simulink model "MIL4L3_SW6_V1_20220211"  (R2018b)
settings: Solver=FixedStepAuto  StartTime=0.0  StopTime=inf  FixedStep=0.001  RelTol=1e-3
PreLoadFcn:
  | A0_MILtest;
undefined symbols (not defined in the file or in its folder): Clb_ICADirect_LaneDisp_StateFive, Clb_ICADirect_LaneDisp_StateFour, Clb_ICADirect_LaneDisp_StateOne, Clb_ICADirect_LaneDisp_StateThree, Clb_ICADirect_LaneDisp_StateTwo, Clb_ICADirect_LaneDisp_StateZero, Clb_ICADirect_LaneDispSW, Clb_ICADirect_TrnLghtsCom_Switch, Clb_ICADirect_TrnLghtsCom_Value, Clb_ICADirect_TrnLghtsCrtl_Inhb, IMAP_Clb_ACU_Driver_Belt, IMAP_Clb_ACU_Driver_Belt_Over, IMAP_Clb_ACU_Passenger_Belt, IMAP_Clb_ACU_Passenger_Belt_Over, IMAP_Clb_ACU_RearLeft_Belt, IMAP_Clb_ACU_RearLeft_Belt_Over, IMAP_Clb_ACU_RearMiddle_Belt, IMAP_Clb_ACU_RearMiddle_Belt_Over, IMAP_Clb_ACU_RearRight_Belt, IMAP_Clb_ACU_RearRight_Belt_Over, IMAP_Clb_AEB_Switch, IMAP_Clb_AEB_Switch_Over, IMAP_Clb_ALC_TLC_Mode, IMAP_Clb_ALC_TLC_Mode_Over, IMAP_Clb_BCM_Battery_Voltage, IMAP_Clb_BCM_Battery_Voltage_Over, IMAP_Clb_BCM_BrakeLamp_State, IMAP_Clb_BCM_BrakeLamp_State_Over, IMAP_Clb_BCM_CHMSL_Status, IMAP_Clb_BCM_CHMSL_Status_Over, IMAP_Clb_BCM_Door_Lock_State, IMAP_Clb_BCM_Door_Lock_State_Over, IMAP_Clb_BCM_FrontWiper_State, IMAP_Clb_BCM_FrontWiper_State_Over, IMAP_Clb_BCM_FrontWiper_Switch, IMAP_Clb_BCM_FrontWiper_Switch_Over, IMAP_Clb_BCM_HazardLamp, IMAP_Clb_BCM_HazardLamp_Over, IMAP_Clb_BCM_HazardLamp_Switch, IMAP_Clb_BCM_HazardLamp_Switch_Over, IMAP_Clb_BCM_HighBeam_State, IMAP_Clb_BCM_HighBeam_State_Over, IMAP_Clb_BCM_Ignition_State, IMAP_Clb_BCM_Ignition_State_Over, IMAP_Clb_BCM_IHBC_Enabled, IMAP_Clb_BCM_IHBC_Enabled_Over, IMAP_Clb_BCM_Left_Light, IMAP_Clb_BCM_Left_Light_Over, IMAP_Clb_BCM_LeftTurn_Switch, IMAP_Clb_BCM_LeftTurn_Switch_Over, IMAP_Clb_BCM_LF_Door_State, IMAP_Clb_BCM_LF_Door_State_Over, IMAP_Clb_BCM_LowBeam_State, IMAP_Clb_BCM_LowBeam_State_Over, IMAP_Clb_BCM_LR_Door_State, IMAP_Clb_BCM_LR_Door_State_Over, IMAP_Clb_BCM_RF_Door_State, IMAP_Clb_BCM_RF_Door_State_Over, IMAP_Clb_BCM_Right_Light, IMAP_Clb_BCM_Right_Light_Over ... (+547)
libraries: CarMaker4SL x2153, simulink x292, dspstat3 x3, canmsglib x2, simulink_extras x1
(part 24 of 52)

== system MIL4L3_SW6_V1_20220211/CarMaker/VehicleControl/Data Inport/SDFA-L3/Subsystem215 ==
  BusCreator : BusCreator  Inputs=24
  Ground{,1..19} (20 alike) : Ground
  Read CM Dict : CarMaker4SL/Read CM Dict  xname=User.IO.Out.ObjectID_00  xsync=off
  Read CM Dict1 : CarMaker4SL/Read CM Dict  xname=User.IO.Out.ObjectID_01  xsync=off
  Read CM Dict2 : CarMaker4SL/Read CM Dict  xname=User.IO.Out.ObjectID_02  xsync=off
  Read CM Dict3 : CarMaker4SL/Read CM Dict  xname=User.IO.Out.ObjectID_03  xsync=off
  ObjectID : Outport
  wires:
  Ground12/1 -> BusCreator/21
  Ground16/1 -> BusCreator/19
  Ground14/1 -> BusCreator/17
  Ground2/1 -> BusCreator/7
  Read CM Dict1/1 -> BusCreator/2
  Ground6/1 -> BusCreator/11
  Read CM Dict2/1 -> BusCreator/3
  Ground10/1 -> BusCreator/15
  Read CM Dict/1 -> BusCreator/1
  Ground17/1 -> BusCreator/20
  Ground4/1 -> BusCreator/9
  Ground13/1 -> BusCreator/22
  Ground/1 -> BusCreator/5
  Ground1/1 -> BusCreator/6
  Ground15/1 -> BusCreator/18
  Ground7/1 -> BusCreator/12
  Ground8/1 -> BusCreator/13
  Ground11/1 -> BusCreator/16
  BusCreator/1 -> ObjectID/1
  Ground9/1 -> BusCreator/14
  Ground3/1 -> BusCreator/8
  Ground5/1 -> BusCreator/10
  Ground18/1 -> BusCreator/23
  Ground19/1 -> BusCreator/24
  Read CM Dict3/1 -> BusCreator/4

== system MIL4L3_SW6_V1_20220211/CarMaker/VehicleControl/Data Inport/SDFA-L3/Subsystem216 ==
  Bus Creator : BusCreator  Inputs=20
  Ground{,1..15} (16 alike) : Ground
  Read CM Dict : CarMaker4SL/Read CM Dict  xname=User.IO.Out.IFC_obj01_Width  xsync=off
  Read CM Dict1 : CarMaker4SL/Read CM Dict  xname=User.IO.Out.IFC_obj02_Width  xsync=off
  Read CM Dict2 : CarMaker4SL/Read CM Dict  xname=User.IO.Out.IFC_obj03_Width  xsync=off
  Read CM Dict3 : CarMaker4SL/Read CM Dict  xname=User.IO.Out.IFC_obj04_Width  xsync=off
  obj_Width : Outport
  wires:
  Bus Creator/1 -> obj_Width/1
  Ground15/1 -> Bus Creator/20
  Ground11/1 -> Bus Creator/16
  Ground14/1 -> Bus Creator/19
  Ground12/1 -> Bus Creator/17
  Ground3/1 -> Bus Creator/8
  Ground1/1 -> Bus Creator/6
  Read CM Dict1/1 -> Bus Creator/2
  Read CM Dict/1 -> Bus Creator/1
  Ground6/1 -> Bus Creator/11
  Ground10/1 -> Bus Creator/15
  Ground13/1 -> Bus Creator/18
  Ground2/1 -> Bus Creator/7
  Ground/1 -> Bus Creator/5
  Ground7/1 -> Bus Creator/12
  Read CM Dict3/1 -> Bus Creator/4
  Ground4/1 -> Bus Creator/9
  Ground9/1 -> Bus Creator/14
  Ground5/1 -> Bus Creator/10
  Ground8/1 -> Bus Creator/13
  Read CM Dict2/1 -> Bus Creator/3

== system MIL4L3_SW6_V1_20220211/CarMaker/VehicleControl/Data Inport/SDFA-L3/Subsystem217 ==
  Bus Creator : BusCreator  Inputs=20
  Ground{,1..15} (16 alike) : Ground
  Read CM Dict : CarMaker4SL/Read CM Dict  xname=User.IO.Out.IFC_obj01_TypeProb  xsync=off
  Read CM Dict1 : CarMaker4SL/Read CM Dict  xname=User.IO.Out.IFC_obj02_TypeProb  xsync=off
  Read CM Dict2 : CarMaker4SL/Read CM Dict  xname=User.IO.Out.IFC_obj03_TypeProb  xsync=off
  Read CM Dict3 : CarMaker4SL/Read CM Dict  xname=User.IO.Out.IFC_obj04_TypeProb  xsync=off
  obj_TypeProb : Outport
  wires:
  Bus Creator/1 -> obj_TypeProb/1
  Ground15/1 -> Bus Creator/20
  Ground11/1 -> Bus Creator/16
  Ground14/1 -> Bus Creator/19
  Ground12/1 -> Bus Creator/17
  Ground3/1 -> Bus Creator/8
  Ground1/1 -> Bus Creator/6
  Read CM Dict1/1 -> Bus Creator/2
  Read CM Dict/1 -> Bus Creator/1
  Ground6/1 -> Bus Creator/11
  Ground10/1 -> Bus Creator/15
  Ground13/1 -> Bus Creator/18
  Ground2/1 -> Bus Creator/7
  Ground/1 -> Bus Creator/5
  Ground7/1 -> Bus Creator/12
  Read CM Dict3/1 -> Bus Creator/4
  Ground4/1 -> Bus Creator/9
  Ground9/1 -> Bus Creator/14
  Ground5/1 -> Bus Creator/10
  Ground8/1 -> Bus Creator/13
  Read CM Dict2/1 -> Bus Creator/3

== system MIL4L3_SW6_V1_20220211/CarMaker/VehicleControl/Data Inport/SDFA-L3/Subsystem218 ==
  Bus Creator : BusCreator  Inputs=20
  Ground{,1..15} (16 alike) : Ground
  Read CM Dict : CarMaker4SL/Read CM Dict  xname=User.IO.Out.IFC_obj01_Height  xsync=off
  Read CM Dict1 : CarMaker4SL/Read CM Dict  xname=User.IO.Out.IFC_obj02_Height  xsync=off
  Read CM Dict2 : CarMaker4SL/Read CM Dict  xname=User.IO.Out.IFC_obj03_Height  xsync=off
  Read CM Dict3 : CarMaker4SL/Read CM Dict  xname=User.IO.Out.IFC_obj04_Height  xsync=off
  obj_Height : Outport
  wires:
  Bus Creator/1 -> obj_Height/1
  Ground15/1 -> Bus Creator/20
  Ground11/1 -> Bus Creator/16
  Ground14/1 -> Bus Creator/19
  Ground12/1 -> Bus Creator/17
  Ground3/1 -> Bus Creator/8
  Ground1/1 -> Bus Creator/6
  Read CM Dict1/1 -> Bus Creator/2
  Read CM Dict/1 -> Bus Creator/1
  Ground6/1 -> Bus Creator/11
  Ground10/1 -> Bus Creator/15
  Ground13/1 -> Bus Creator/18
  Ground2/1 -> Bus Creator/7
  Ground/1 -> Bus Creator/5
  Ground7/1 -> Bus Creator/12
  Read CM Dict3/1 -> Bus Creator/4
  Ground4/1 -> Bus Creator/9
  Ground9/1 -> Bus Creator/14
  Ground5/1 -> Bus Creator/10
  Ground8/1 -> Bus Creator/13
  Read CM Dict2/1 -> Bus Creator/3

== system MIL4L3_SW6_V1_20220211/CarMaker/VehicleControl/Data Inport/SDFA-L3/Subsystem219 ==
  BusCreator : BusCreator  Inputs=24
  Ground{,1..19} (20 alike) : Ground
  Read CM Dict : CarMaker4SL/Read CM Dict  xname=User.IO.Out.YawAngle_00  xsync=off
  Read CM Dict1 : CarMaker4SL/Read CM Dict  xname=User.IO.Out.YawAngle_01  xsync=off
  Read CM Dict2 : CarMaker4SL/Read CM Dict  xname=User.IO.Out.YawAngle_02  xsync=off
  Read CM Dict3 : CarMaker4SL/Read CM Dict  xname=User.IO.Out.YawAngle_03  xsync=off
  YawAngle : Outport
  wires:
  Ground12/1 -> BusCreator/21
  Ground16/1 -> BusCreator/19
  Ground14/1 -> BusCreator/17
  Ground2/1 -> BusCreator/7
  Read CM Dict1/1 -> BusCreator/2
  Ground6/1 -> BusCreator/11
  Read CM Dict2/1 -> BusCreator/3
  Ground10/1 -> BusCreator/15
  Read CM Dict/1 -> BusCreator/1
  Ground17/1 -> BusCreator/20
  Ground4/1 -> BusCreator/9
  Ground13/1 -> BusCreator/22
  Ground/1 -> BusCreator/5
  Ground1/1 -> BusCreator/6
  Ground15/1 -> BusCreator/18
  Ground7/1 -> BusCreator/12
  Ground8/1 -> BusCreator/13
  Ground11/1 -> BusCreator/16
  BusCreator/1 -> YawAngle/1
  Ground9/1 -> BusCreator/14
  Ground3/1 -> BusCreator/8
  Ground5/1 -> BusCreator/10
  Ground18/1 -> BusCreator/23
  Ground19/1 -> BusCreator/24
  Read CM Dict3/1 -> BusCreator/4

== system MIL4L3_SW6_V1_20220211/CarMaker/VehicleControl/Data Inport/SDFA-L3/Subsystem220 ==
  Bus Creator : BusCreator  Inputs=20
  Ground{,1..15} (16 alike) : Ground
  Read CM Dict : CarMaker4SL/Read CM Dict  xname=User.IO.Out.IFC_obj01_Length  xsync=off
  Read CM Dict1 : CarMaker4SL/Read CM Dict  xname=User.IO.Out.IFC_obj02_Length  xsync=off
  Read CM Dict2 : CarMaker4SL/Read CM Dict  xname=User.IO.Out.IFC_obj03_Length  xsync=off
  Read CM Dict3 : CarMaker4SL/Read CM Dict  xname=User.IO.Out.IFC_obj04_Length  xsync=off
  obj_Length : Outport
  wires:
  Bus Creator/1 -> obj_Length/1
  Ground15/1 -> Bus Creator/20
  Ground11/1 -> Bus Creator/16
  Ground14/1 -> Bus Creator/19
  Ground12/1 -> Bus Creator/17
  Ground3/1 -> Bus Creator/8
  Ground1/1 -> Bus Creator/6
  Read CM Dict1/1 -> Bus Creator/2
  Read CM Dict/1 -> Bus Creator/1
  Ground6/1 -> Bus Creator/11
  Ground10/1 -> Bus Creator/15
  Ground13/1 -> Bus Creator/18
  Ground2/1 -> Bus Creator/7
  Ground/1 -> Bus Creator/5
  Ground7/1 -> Bus Creator/12
  Read CM Dict3/1 -> Bus Creator/4
  Ground4/1 -> Bus Creator/9
  Ground9/1 -> Bus Creator/14
  Ground5/1 -> Bus Creator/10
  Ground8/1 -> Bus Creator/13
  Read CM Dict2/1 -> Bus Creator/3

== system MIL4L3_SW6_V1_20220211/CarMaker/VehicleControl/Data Inport/SDFA-L3/Subsystem221 ==
  BusCreator : BusCreator  Inputs=24
  Ground{,1..19} (20 alike) : Ground
  Read CM Dict : CarMaker4SL/Read CM Dict  xname=User.IO.Out.MovementStatus_00  xsync=off
  Read CM Dict1 : CarMaker4SL/Read CM Dict  xname=User.IO.Out.MovementStatus_01  xsync=off
  Read CM Dict2 : CarMaker4SL/Read CM Dict  xname=User.IO.Out.MovementStatus_02  xsync=off
  Read CM Dict3 : CarMaker4SL/Read CM Dict  xname=User.IO.Out.MovementStatus_03  xsync=off
  MovementStatus : Outport
  wires:
  Ground12/1 -> BusCreator/21
  Ground16/1 -> BusCreator/19
  Ground14/1 -> BusCreator/17
  Ground2/1 -> BusCreator/7
  Read CM Dict1/1 -> BusCreator/2
  Ground6/1 -> BusCreator/11
  Read CM Dict2/1 -> BusCreator/3
  Ground10/1 -> BusCreator/15
  Read CM Dict/1 -> BusCreator/1
  Ground17/1 -> BusCreator/20
  Ground4/1 -> BusCreator/9
  Ground13/1 -> BusCreator/22
  Ground/1 -> BusCreator/5
  Ground1/1 -> BusCreator/6
  Ground15/1 -> BusCreator/18
  Ground7/1 -> BusCreator/12
  Ground8/1 -> BusCreator/13
  Ground11/1 -> BusCreator/16
  BusCreator/1 -> MovementStatus/1
  Ground9/1 -> BusCreator/14
  Ground3/1 -> BusCreator/8
  Ground5/1 -> BusCreator/10
  Ground18/1 -> BusCreator/23
  Ground19/1 -> BusCreator/24
  Read CM Dict3/1 -> BusCreator/4

== system MIL4L3_SW6_V1_20220211/CarMaker/VehicleControl/Data Inport/SDFA-L3/Subsystem222 ==
  BusCreator : BusCreator  Inputs=24
  Ground{,1..19} (20 alike) : Ground
  Read CM Dict : CarMaker4SL/Read CM Dict  xname=User.IO.Out.MeasurementStatus_00  xsync=off
  Read CM Dict1 : CarMaker4SL/Read CM Dict  xname=User.IO.Out.MeasurementStatus_01  xsync=off
  Read CM Dict2 : CarMaker4SL/Read CM Dict  xname=User.IO.Out.MeasurementStatus_02  xsync=off
  Read CM Dict3 : CarMaker4SL/Read CM Dict  xname=User.IO.Out.MeasurementStatus_03  xsync=off
  MeasurementStatus : Outport
  wires:
  Ground12/1 -> BusCreator/21
  Ground16/1 -> BusCreator/19
  Ground14/1 -> BusCreator/17
  Ground2/1 -> BusCreator/7
  Read CM Dict1/1 -> BusCreator/2
  Ground6/1 -> BusCreator/11
  Read CM Dict2/1 -> BusCreator/3
  Ground10/1 -> BusCreator/15
  Read CM Dict/1 -> BusCreator/1
  Ground17/1 -> BusCreator/20
  Ground4/1 -> BusCreator/9
  Ground13/1 -> BusCreator/22
  Ground/1 -> BusCreator/5
  Ground1/1 -> BusCreator/6
  Ground15/1 -> BusCreator/18
  Ground7/1 -> BusCreator/12
  Ground8/1 -> BusCreator/13
  Ground11/1 -> BusCreator/16
  BusCreator/1 -> MeasurementStatus/1
  Ground9/1 -> BusCreator/14
  Ground3/1 -> BusCreator/8
  Ground5/1 -> BusCreator/10
  Ground18/1 -> BusCreator/23
  Ground19/1 -> BusCreator/24
  Read CM Dict3/1 -> BusCreator/4

== system MIL4L3_SW6_V1_20220211/CarMaker/VehicleControl/Data Inport/SDFA-L3/Subsystem223 ==
  Bus Creator : BusCreator  Inputs=20
  Ground{,1..15} (16 alike) : Ground
  Read CM Dict : CarMaker4SL/Read CM Dict  xname=User.IO.Out.IFC_obj01_ID  xsync=off
  Read CM Dict1 : CarMaker4SL/Read CM Dict  xname=User.IO.Out.IFC_obj02_ID  xsync=off
  Read CM Dict2 : CarMaker4SL/Read CM Dict  xname=User.IO.Out.IFC_obj03_ID  xsync=off
  Read CM Dict3 : CarMaker4SL/Read CM Dict  xname=User.IO.Out.IFC_obj04_ID  xsync=off
  obj_ID : Outport
  wires:
  Bus Creator/1 -> obj_ID/1
  Ground15/1 -> Bus Creator/20
  Ground11/1 -> Bus Creator/16
  Ground14/1 -> Bus Creator/19
  Ground12/1 -> Bus Creator/17
  Ground3/1 -> Bus Creator/8
  Ground1/1 -> Bus Creator/6
  Read CM Dict1/1 -> Bus Creator/2
  Read CM Dict/1 -> Bus Creator/1
  Ground6/1 -> Bus Creator/11
  Ground10/1 -> Bus Creator/15
  Ground13/1 -> Bus Creator/18
  Ground2/1 -> Bus Creator/7
  Ground/1 -> Bus Creator/5
  Ground7/1 -> Bus Creator/12
  Read CM Dict3/1 -> Bus Creator/4
  Ground4/1 -> Bus Creator/9
  Ground9/1 -> Bus Creator/14
  Ground5/1 -> Bus Creator/10
  Ground8/1 -> Bus Creator/13
  Read CM Dict2/1 -> Bus Creator/3

== system MIL4L3_SW6_V1_20220211/CarMaker/VehicleControl/Data Inport/SDFA-L3/Subsystem224 ==
  Bus Creator : BusCreator  Inputs=20
  Ground{,1..15} (16 alike) : Ground
  Read CM Dict : CarMaker4SL/Read CM Dict  xname=User.IO.Out.IFC_obj01_Heading  xsync=off
  Read CM Dict1 : CarMaker4SL/Read CM Dict  xname=User.IO.Out.IFC_obj02_Heading  xsync=off
  Read CM Dict2 : CarMaker4SL/Read CM Dict  xname=User.IO.Out.IFC_obj03_Heading  xsync=off
  Read CM Dict3 : CarMaker4SL/Read CM Dict  xname=User.IO.Out.IFC_obj04_Heading  xsync=off
  obj_Heading : Outport
  wires:
  Bus Creator/1 -> obj_Heading/1
  Ground15/1 -> Bus Creator/20
  Ground11/1 -> Bus Creator/16
  Ground14/1 -> Bus Creator/19
  Ground12/1 -> Bus Creator/17
  Ground3/1 -> Bus Creator/8
  Ground1/1 -> Bus Creator/6
  Read CM Dict1/1 -> Bus Creator/2
  Read CM Dict/1 -> Bus Creator/1
  Ground6/1 -> Bus Creator/11
  Ground10/1 -> Bus Creator/15
  Ground13/1 -> Bus Creator/18
  Ground2/1 -> Bus Creator/7
  Ground/1 -> Bus Creator/5
  Ground7/1 -> Bus Creator/12
  Read CM Dict3/1 -> Bus Creator/4
  Ground4/1 -> Bus Creator/9
  Ground9/1 -> Bus Creator/14
  Ground5/1 -> Bus Creator/10
  Ground8/1 -> Bus Creator/13
  Read CM Dict2/1 -> Bus Creator/3

== system MIL4L3_SW6_V1_20220211/CarMaker/VehicleControl/Data Inport/SDFA-L3/Subsystem225 ==
  BusCreator : BusCreator  Inputs=24
  Ground{,1..19} (20 alike) : Ground
  Read CM Dict : CarMaker4SL/Read CM Dict  xname=User.IO.Out.ExistenceProb_00  xsync=off
  Read CM Dict1 : CarMaker4SL/Read CM Dict  xname=User.IO.Out.ExistenceProb_01  xsync=off
  Read CM Dict2 : CarMaker4SL/Read CM Dict  xname=User.IO.Out.ExistenceProb_02  xsync=off
  Read CM Dict3 : CarMaker4SL/Read CM Dict  xname=User.IO.Out.ExistenceProb_03  xsync=off
  ExistenceProb : Outport
  wires:
  Ground12/1 -> BusCreator/21
  Ground16/1 -> BusCreator/19
  Ground14/1 -> BusCreator/17
  Ground2/1 -> BusCreator/7
  Read CM Dict1/1 -> BusCreator/2
  Ground6/1 -> BusCreator/11
  Read CM Dict2/1 -> BusCreator/3
  Ground10/1 -> BusCreator/15
  Read CM Dict/1 -> BusCreator/1
  Ground17/1 -> BusCreator/20
  Ground4/1 -> BusCreator/9
  Ground13/1 -> BusCreator/22
  Ground/1 -> BusCreator/5
  Ground1/1 -> BusCreator/6
  Ground15/1 -> BusCreator/18
  Ground7/1 -> BusCreator/12
  Ground8/1 -> BusCreator/13
  Ground11/1 -> BusCreator/16
  BusCreator/1 -> ExistenceProb/1
  Ground9/1 -> BusCreator/14
  Ground3/1 -> BusCreator/8
  Ground5/1 -> BusCreator/10
  Ground18/1 -> BusCreator/23
  Ground19/1 -> BusCreator/24
  Read CM Dict3/1 -> BusCreator/4

== system MIL4L3_SW6_V1_20220211/CarMaker/VehicleControl/Data Inport/SDFA-L3/Subsystem226 ==
  Bus Creator : BusCreator  Inputs=20
  Ground{,1..15} (16 alike) : Ground
  Read CM Dict : CarMaker4SL/Read CM Dict  xname=User.IO.Out.IFC_obj01_TTIPC  xsync=off
  Read CM Dict1 : CarMaker4SL/Read CM Dict  xname=User.IO.Out.IFC_obj02_TTIPC  xsync=off
  Read CM Dict2 : CarMaker4SL/Read CM Dict  xname=User.IO.Out.IFC_obj03_TTIPC  xsync=off
  Read CM Dict3 : CarMaker4SL/Read CM Dict  xname=User.IO.Out.IFC_obj04_TTIPC  xsync=off
  obj_TTIPC : Outport
  wires:
  Bus Creator/1 -> obj_TTIPC/1
  Ground15/1 -> Bus Creator/20
  Ground11/1 -> Bus Creator/16
  Ground14/1 -> Bus Creator/19
  Ground12/1 -> Bus Creator/17
  Ground3/1 -> Bus Creator/8
  Ground1/1 -> Bus Creator/6
  Read CM Dict1/1 -> Bus Creator/2
  Read CM Dict/1 -> Bus Creator/1
  Ground6/1 -> Bus Creator/11
  Ground10/1 -> Bus Creator/15
  Ground13/1 -> Bus Creator/18
  Ground2/1 -> Bus Creator/7
  Ground/1 -> Bus Creator/5
  Ground7/1 -> Bus Creator/12
  Read CM Dict3/1 -> Bus Creator/4
  Ground4/1 -> Bus Creator/9
  Ground9/1 -> Bus Creator/14
  Ground5/1 -> Bus Creator/10
  Ground8/1 -> Bus Creator/13
  Read CM Dict2/1 -> Bus Creator/3

== system MIL4L3_SW6_V1_20220211/CarMaker/VehicleControl/Data Inport/SDFA-L3/Subsystem227 ==
  Bus Creator : BusCreator  Inputs=20
  Ground{,1..15} (16 alike) : Ground
  Read CM Dict : CarMaker4SL/Read CM Dict  xname=User.IO.Out.IFC_obj01_Measured  xsync=off
  Read CM Dict1 : CarMaker4SL/Read CM Dict  xname=User.IO.Out.IFC_obj02_Measured  xsync=off
  Read CM Dict2 : CarMaker4SL/Read CM Dict  xname=User.IO.Out.IFC_obj03_Measured  xsync=off
  Read CM Dict3 : CarMaker4SL/Read CM Dict  xname=User.IO.Out.IFC_obj04_Measured  xsync=off
  obj_Measured : Outport
  wires:
  Bus Creator/1 -> obj_Measured/1
  Ground15/1 -> Bus Creator/20
  Ground11/1 -> Bus Creator/16
  Ground14/1 -> Bus Creator/19
  Ground12/1 -> Bus Creator/17
  Ground3/1 -> Bus Creator/8
  Ground1/1 -> Bus Creator/6
  Read CM Dict1/1 -> Bus Creator/2
  Read CM Dict/1 -> Bus Creator/1
  Ground6/1 -> Bus Creator/11
  Ground10/1 -> Bus Creator/15
  Ground13/1 -> Bus Creator/18
  Ground2/1 -> Bus Creator/7
  Ground/1 -> Bus Creator/5
  Ground7/1 -> Bus Creator/12
  Read CM Dict3/1 -> Bus Creator/4
  Ground4/1 -> Bus Creator/9
  Ground9/1 -> Bus Creator/14
  Ground5/1 -> Bus Creator/10
  Ground8/1 -> Bus Creator/13
  Read CM Dict2/1 -> Bus Creator/3

== system MIL4L3_SW6_V1_20220211/CarMaker/VehicleControl/Data Inport/SDFA-L3/Subsystem228 ==
  Bus Creator : BusCreator  Inputs=20
  Ground{,1..15} (16 alike) : Ground
  Read CM Dict : CarMaker4SL/Read CM Dict  xname=User.IO.Out.IFC_obj01_Type  xsync=off
  Read CM Dict1 : CarMaker4SL/Read CM Dict  xname=User.IO.Out.IFC_obj02_Type  xsync=off
  Read CM Dict2 : CarMaker4SL/Read CM Dict  xname=User.IO.Out.IFC_obj03_Type  xsync=off
  Read CM Dict3 : CarMaker4SL/Read CM Dict  xname=User.IO.Out.IFC_obj04_Type  xsync=off
  obj_Type : Outport
  wires:
  Bus Creator/1 -> obj_Type/1
  Ground15/1 -> Bus Creator/20
  Ground11/1 -> Bus Creator/16
  Ground14/1 -> Bus Creator/19
  Ground12/1 -> Bus Creator/17
  Ground3/1 -> Bus Creator/8
  Ground1/1 -> Bus Creator/6
  Read CM Dict1/1 -> Bus Creator/2
  Read CM Dict/1 -> Bus Creator/1
  Ground6/1 -> Bus Creator/11
  Ground10/1 -> Bus Creator/15
  Ground13/1 -> Bus Creator/18
  Ground2/1 -> Bus Creator/7
  Ground/1 -> Bus Creator/5
  Ground7/1 -> Bus Creator/12
  Read CM Dict3/1 -> Bus Creator/4
  Ground4/1 -> Bus Creator/9
  Ground9/1 -> Bus Creator/14
  Ground5/1 -> Bus Creator/10
  Ground8/1 -> Bus Creator/13
  Read CM Dict2/1 -> Bus Creator/3

== system MIL4L3_SW6_V1_20220211/CarMaker/VehicleControl/Data Inport/SDFA-L3/Subsystem230 ==
  BusCreator : BusCreator  Inputs=24
  Ground{,1..19} (20 alike) : Ground
  Read CM Dict : CarMaker4SL/Read CM Dict  xname=User.IO.Out.T00.RelativeLatVelo  xsync=off
  Read CM Dict1 : CarMaker4SL/Read CM Dict  xname=User.IO.Out.T01.RelativeLatVelo  xsync=off
  Read CM Dict2 : CarMaker4SL/Read CM Dict  xname=User.IO.Out.T02.RelativeLatVelo  xsync=off
  Read CM Dict3 : CarMaker4SL/Read CM Dict  xname=User.IO.Out.T03.RelativeLatVelo  xsync=off
  RelativeLatVelo : Outport
  wires:
  Ground12/1 -> BusCreator/21
  Ground16/1 -> BusCreator/19
  Ground14/1 -> BusCreator/17
  Ground2/1 -> BusCreator/7
  Read CM Dict1/1 -> BusCreator/2
  Ground6/1 -> BusCreator/11
  Read CM Dict2/1 -> BusCreator/3
  Ground10/1 -> BusCreator/15
  Read CM Dict/1 -> BusCreator/1
  Ground17/1 -> BusCreator/20
  Ground4/1 -> BusCreator/9
  Ground13/1 -> BusCreator/22
  Ground/1 -> BusCreator/5
  Ground1/1 -> BusCreator/6
  Ground15/1 -> BusCreator/18
  Ground7/1 -> BusCreator/12
  Ground8/1 -> BusCreator/13
  Ground11/1 -> BusCreator/16
  BusCreator/1 -> RelativeLatVelo/1
  Ground9/1 -> BusCreator/14
  Ground3/1 -> BusCreator/8
  Ground5/1 -> BusCreator/10
  Ground18/1 -> BusCreator/23
  Ground19/1 -> BusCreator/24
  Read CM Dict3/1 -> BusCreator/4

== system MIL4L3_SW6_V1_20220211/CarMaker/VehicleControl/Data Inport/SDFA-L3/Subsystem232 ==
  BusCreator : BusCreator  Inputs=24
  Ground{,1..19} (20 alike) : Ground
  Read CM Dict : CarMaker4SL/Read CM Dict  xname=User.IO.Out.ClassProbValue_00  xsync=off
  Read CM Dict1 : CarMaker4SL/Read CM Dict  xname=User.IO.Out.ClassProbValue_01  xsync=off
  Read CM Dict2 : CarMaker4SL/Read CM Dict  xname=User.IO.Out.ClassProbValue_02  xsync=off
  Read CM Dict3 : CarMaker4SL/Read CM Dict  xname=User.IO.Out.ClassProbValue_03  xsync=off
  ClassProbValue : Outport
  wires:
  Read CM Dict3/1 -> BusCreator/4
  Ground19/1 -> BusCreator/24
  Ground18/1 -> BusCreator/23
  Ground5/1 -> BusCreator/10
  Ground3/1 -> BusCreator/8
  Ground9/1 -> BusCreator/14
  BusCreator/1 -> ClassProbValue/1
  Ground11/1 -> BusCreator/16
  Ground8/1 -> BusCreator/13
  Ground7/1 -> BusCreator/12
  Ground15/1 -> BusCreator/18
  Ground1/1 -> BusCreator/6
  Ground/1 -> BusCreator/5
  Ground13/1 -> BusCreator/22
  Ground4/1 -> BusCreator/9
  Ground17/1 -> BusCreator/20
  Read CM Dict/1 -> BusCreator/1
  Ground10/1 -> BusCreator/15
  Read CM Dict2/1 -> BusCreator/3
  Ground6/1 -> BusCreator/11
  Read CM Dict1/1 -> BusCreator/2
  Ground2/1 -> BusCreator/7
  Ground14/1 -> BusCreator/17
  Ground16/1 -> BusCreator/19
  Ground12/1 -> BusCreator/21

== system MIL4L3_SW6_V1_20220211/CarMaker/VehicleControl/Data Inport/SDFA-L3/Subsystem239 ==
  BusCreator : BusCreator  Inputs=24
  Ground{,1..19} (20 alike) : Ground
  Read CM Dict : CarMaker4SL/Read CM Dict  xname=User.IO.Out.T00.RelativeLongVelo  xsync=off
  Read CM Dict1 : CarMaker4SL/Read CM Dict  xname=User.IO.Out.T01.RelativeLongVelo  xsync=off
  Read CM Dict2 : CarMaker4SL/Read CM Dict  xname=User.IO.Out.T02.RelativeLongVelo  xsync=off
  Read CM Dict3 : CarMaker4SL/Read CM Dict  xname=User.IO.Out.T03.RelativeLongVelo  xsync=off
  RelLongVel : Outport
  wires:
  Read CM Dict3/1 -> BusCreator/4
  Ground5/1 -> BusCreator/10
  BusCreator/1 -> RelLongVel/1
  Ground18/1 -> BusCreator/23
  Ground19/1 -> BusCreator/24
  Ground8/1 -> BusCreator/13
  Ground3/1 -> BusCreator/8
  Ground9/1 -> BusCreator/14
  Ground15/1 -> BusCreator/18
  Ground1/1 -> BusCreator/6
  Ground/1 -> BusCreator/5
  Ground11/1 -> BusCreator/16
  Ground4/1 -> BusCreator/9
  Ground10/1 -> BusCreator/15
  Ground6/1 -> BusCreator/11
  Ground13/1 -> BusCreator/22
  Read CM Dict2/1 -> BusCreator/3
  Read CM Dict1/1 -> BusCreator/2
  Ground17/1 -> BusCreator/20
  Read CM Dict/1 -> BusCreator/1
  Ground14/1 -> BusCreator/17
  Ground16/1 -> BusCreator/19
  Ground12/1 -> BusCreator/21
  Ground7/1 -> BusCreator/12
  Ground2/1 -> BusCreator/7

== system MIL4L3_SW6_V1_20220211/CarMaker/VehicleControl/Data Inport/SDFA-L3/Subsystem255 ==
  BusCreator : BusCreator  Inputs=24
  Constant{1..4} (4 alike) : Constant  Value=0.01
  Ground{,1..19} (20 alike) : Ground
  AbsoluteLongVeloSTD : Outport
  wires:
  Constant4/1 -> BusCreator/4
  Ground19/1 -> BusCreator/24
  Ground18/1 -> BusCreator/23
  Ground5/1 -> BusCreator/10
  Ground3/1 -> BusCreator/8
  Ground9/1 -> BusCreator/14
  BusCreator/1 -> AbsoluteLongVeloSTD/1
  Ground11/1 -> BusCreator/16
  Ground8/1 -> BusCreator/13
  Ground7/1 -> BusCreator/12
  Ground15/1 -> BusCreator/18
  Ground1/1 -> BusCreator/6
  Ground/1 -> BusCreator/5
  Ground13/1 -> BusCreator/22
  Ground4/1 -> BusCreator/9
  Ground17/1 -> BusCreator/20
  Constant2/1 -> BusCreator/1
  Ground10/1 -> BusCreator/15
  Constant3/1 -> BusCreator/3
  Ground6/1 -> BusCreator/11
  Constant1/1 -> BusCreator/2
  Ground2/1 -> BusCreator/7
  Ground14/1 -> BusCreator/17
  Ground16/1 -> BusCreator/19
  Ground12/1 -> BusCreator/21

== system MIL4L3_SW6_V1_20220211/CarMaker/VehicleControl/Data Inport/SDFA-L3/Subsystem261 ==
  BusCreator : BusCreator  Inputs=24
  Ground{,1..19} (20 alike) : Ground
  Read CM Dict : CarMaker4SL/Read CM Dict  xname=User.IO.Out.T00.RelativeLatAcc  xsync=off
  Read CM Dict1 : CarMaker4SL/Read CM Dict  xname=User.IO.Out.T01.RelativeLatAcc  xsync=off
  Read CM Dict2 : CarMaker4SL/Read CM Dict  xname=User.IO.Out.T02.RelativeLatAcc  xsync=off
  Read CM Dict3 : CarMaker4SL/Read CM Dict  xname=User.IO.Out.T03.RelativeLatAcc  xsync=off
  RelativeLatAcc : Outport
  wires:
  Ground12/1 -> BusCreator/21
  Ground16/1 -> BusCreator/19
  Ground14/1 -> BusCreator/17
  Ground2/1 -> BusCreator/7
  Read CM Dict1/1 -> BusCreator/2
  Ground6/1 -> BusCreator/11
  Read CM Dict2/1 -> BusCreator/3
  Ground10/1 -> BusCreator/15
  Read CM Dict/1 -> BusCreator/1
  Ground17/1 -> BusCreator/20
  Ground4/1 -> BusCreator/9
  Ground13/1 -> BusCreator/22
  Ground/1 -> BusCreator/5
  Ground1/1 -> BusCreator/6
  Ground15/1 -> BusCreator/18
  Ground7/1 -> BusCreator/12
  Ground8/1 -> BusCreator/13
  Ground11/1 -> BusCreator/16
  BusCreator/1 -> RelativeLatAcc/1
  Ground9/1 -> BusCreator/14
  Ground3/1 -> BusCreator/8
  Ground5/1 -> BusCreator/10
  Ground18/1 -> BusCreator/23
  Ground19/1 -> BusCreator/24
  Read CM Dict3/1 -> BusCreator/4

== system MIL4L3_SW6_V1_20220211/CarMaker/VehicleControl/Data Inport/SDFA-L3/Subsystem272 ==
  BusCreator : BusCreator  Inputs=24
  Ground{,1..19} (20 alike) : Ground
  Read CM Dict : CarMaker4SL/Read CM Dict  xname=User.IO.Out.T00.RelativeLongAcc  xsync=off
  Read CM Dict1 : CarMaker4SL/Read CM Dict  xname=User.IO.Out.T01.RelativeLongAcc  xsync=off
  Read CM Dict2 : CarMaker4SL/Read CM Dict  xname=User.IO.Out.T02.RelativeLongAcc  xsync=off
  Read CM Dict3 : CarMaker4SL/Read CM Dict  xname=User.IO.Out.T03.RelativeLongAcc  xsync=off
  RelativeLongAcc : Outport
  wires:
  Ground12/1 -> BusCreator/21
  Ground16/1 -> BusCreator/19
  Ground14/1 -> BusCreator/17
  Ground2/1 -> BusCreator/7
  Read CM Dict1/1 -> BusCreator/2
  Ground6/1 -> BusCreator/11
  Read CM Dict2/1 -> BusCreator/3
  Ground10/1 -> BusCreator/15
  Read CM Dict/1 -> BusCreator/1
  Ground17/1 -> BusCreator/20
  Ground4/1 -> BusCreator/9
  Ground13/1 -> BusCreator/22
  Ground/1 -> BusCreator/5
  Ground1/1 -> BusCreator/6
  Ground15/1 -> BusCreator/18
  Ground7/1 -> BusCreator/12
  Ground8/1 -> BusCreator/13
  Ground11/1 -> BusCreator/16
  BusCreator/1 -> RelativeLongAcc/1
  Ground9/1 -> BusCreator/14
  Ground3/1 -> BusCreator/8
  Ground5/1 -> BusCreator/10
  Ground18/1 -> BusCreator/23
  Ground19/1 -> BusCreator/24
  Read CM Dict3/1 -> BusCreator/4

== system MIL4L3_SW6_V1_20220211/CarMaker/VehicleControl/Data Inport/SDFA-L3/Subsystem283 ==
  BusCreator : BusCreator  Inputs=24
  Ground{,1..19} (20 alike) : Ground
  Read CM Dict : CarMaker4SL/Read CM Dict  xname=User.IO.Out.AbsoluteLongVelo_00  xsync=off
  Read CM Dict1 : CarMaker4SL/Read CM Dict  xname=User.IO.Out.AbsoluteLongVelo_01  xsync=off
  Read CM Dict2 : CarMaker4SL/Read CM Dict  xname=User.IO.Out.AbsoluteLongVelo_02  xsync=off
  Read CM Dict3 : CarMaker4SL/Read CM Dict  xname=User.IO.Out.AbsoluteLongVelo_03  xsync=off
  AbsoluteLongVelo : Outport
  wires:
  Ground12/1 -> BusCreator/21
  Ground16/1 -> BusCreator/19
  Ground14/1 -> BusCreator/17
  Ground2/1 -> BusCreator/7
  Read CM Dict1/1 -> BusCreator/2
  Ground6/1 -> BusCreator/11
  Read CM Dict2/1 -> BusCreator/3
  Ground10/1 -> BusCreator/15
  Read CM Dict/1 -> BusCreator/1
  Ground17/1 -> BusCreator/20
  Ground4/1 -> BusCreator/9
  Ground13/1 -> BusCreator/22
  Ground/1 -> BusCreator/5
  Ground1/1 -> BusCreator/6
  Ground15/1 -> BusCreator/18
  Ground7/1 -> BusCreator/12
  Ground8/1 -> BusCreator/13
  Ground11/1 -> BusCreator/16
  BusCreator/1 -> AbsoluteLongVelo/1
  Ground9/1 -> BusCreator/14
  Ground3/1 -> BusCreator/8
  Ground5/1 -> BusCreator/10
  Ground18/1 -> BusCreator/23
  Ground19/1 -> BusCreator/24
  Read CM Dict3/1 -> BusCreator/4

== system MIL4L3_SW6_V1_20220211/CarMaker/VehicleControl/Data Inport/SDFA-L3/Subsystem3 ==
  BusCreator : BusCreator  Inputs=24
  Ground{,1..19} (20 alike) : Ground
  Read CM Dict : CarMaker4SL/Read CM Dict  xname=User.IO.Out.ReferencePoint_00  xsync=off
  Read CM Dict1 : CarMaker4SL/Read CM Dict  xname=User.IO.Out.ReferencePoint_01  xsync=off
  Read CM Dict2 : CarMaker4SL/Read CM Dict  xname=User.IO.Out.ReferencePoint_02  xsync=off
  Read CM Dict3 : CarMaker4SL/Read CM Dict  xname=User.IO.Out.ReferencePoint_03  xsync=off
  ReferencePoint : Outport
  wires:
  Ground12/1 -> BusCreator/21
  Ground16/1 -> BusCreator/19
  Ground14/1 -> BusCreator/17
  Ground2/1 -> BusCreator/7
  Read CM Dict1/1 -> BusCreator/2
  Ground6/1 -> BusCreator/11
  Read CM Dict2/1 -> BusCreator/3
  Ground10/1 -> BusCreator/15
  Read CM Dict/1 -> BusCreator/1
  Ground17/1 -> BusCreator/20
  Ground4/1 -> BusCreator/9
  Ground13/1 -> BusCreator/22
  Ground/1 -> BusCreator/5
  Ground1/1 -> BusCreator/6
  Ground15/1 -> BusCreator/18
  Ground7/1 -> BusCreator/12
  Ground8/1 -> BusCreator/13
  Ground11/1 -> BusCreator/16
  BusCreator/1 -> ReferencePoint/1
  Ground9/1 -> BusCreator/14
  Ground3/1 -> BusCreator/8
  Ground5/1 -> BusCreator/10
  Ground18/1 -> BusCreator/23
  Ground19/1 -> BusCreator/24
  Read CM Dict3/1 -> BusCreator/4

== system MIL4L3_SW6_V1_20220211/CarMaker/VehicleControl/Data Inport/SDFA-L3/Subsystem4 ==
  BusCreator : BusCreator  Inputs=20
  Subsystem : Subsystem
  Subsystem1 : Subsystem
  Subsystem10 : Subsystem
  Subsystem11 : Subsystem
  Subsystem12 : Subsystem
  Subsystem13 : Subsystem
  Subsystem14 : Subsystem
  Subsystem15 : Subsystem
  Subsystem16 : Subsystem
  Subsystem17 : Subsystem
  Subsystem18 : Subsystem
  Subsystem19 : Subsystem
  Subsystem2 : Subsystem
  Subsystem3 : Subsystem
  Subsystem4 : Subsystem
  Subsystem5 : Subsystem
  Subsystem6 : Subsystem
  Subsystem7 : Subsystem
  Subsystem8 : Subsystem
  Subsystem9 : Subsystem
  Out1 : Outport
  wires:
  BusCreator/1 -> Out1/1
  Subsystem/1(Out1) -> BusCreator/1
  Subsystem1/1(Out1) -> BusCreator/2
  Subsystem2/1(Out1) -> BusCreator/3
  Subsystem3/1(Out1) -> BusCreator/4
  Subsystem7/1(Out1) -> BusCreator/8
  Subsystem6/1(Out1) -> BusCreator/7
  Subsystem5/1(Out1) -> BusCreator/6
  Subsystem4/1(Out1) -> BusCreator/5
  Subsystem8/1(Out1) -> BusCreator/9
  Subsystem9/1(Out1) -> BusCreator/10
  Subsystem10/1(Out1) -> BusCreator/11
  Subsystem11/1(Out1) -> BusCreator/12
  Subsystem12/1(Out1) -> BusCreator/13
  Subsystem13/1(Out1) -> BusCreator/14
  Subsystem14/1(Out1) -> BusCreator/15
  Subsystem15/1(Out1) -> BusCreator/16
  Subsystem16/1(Out1) -> BusCreator/17
  Subsystem17/1(Out1) -> BusCreator/18
  Subsystem18/1(Out1) -> BusCreator/19
  Subsystem19/1(Out1) -> BusCreator/20

== system MIL4L3_SW6_V1_20220211/CarMaker/VehicleControl/Data Inport/SDFA-L3/Subsystem40 ==
  BusCreator : BusCreator  Inputs=24
  Subsystem : Subsystem  Commented=on
  Subsystem1 : Subsystem  Commented=on
  Subsystem10 : Subsystem
  Subsystem11 : Subsystem
  Subsystem12 : Subsystem
  Subsystem13 : Subsystem
  Subsystem14 : Subsystem
  Subsystem15 : Subsystem
  Subsystem16 : Subsystem
  Subsystem17 : Subsystem
  Subsystem18 : Subsystem
  Subsystem19 : Subsystem
  Subsystem2 : Subsystem  Commented=on
  Subsystem20 : Subsystem
  Subsystem21 : Subsystem
  Subsystem22 : Subsystem
  Subsystem23 : Subsystem
  Subsystem24 : Subsystem
  Subsystem25 : Subsystem
  Subsystem26 : Subsystem
  Subsystem27 : Subsystem
  Subsystem3 : Subsystem  Commented=on
  Subsystem4 : Subsystem
  Subsystem5 : Subsystem
  Subsystem6 : Subsystem
  Subsystem7 : Subsystem
  Subsystem8 : Subsystem
  Subsystem9 : Subsystem
  TimeStamp : Outport
  wires:
  Subsystem21/1(Out1) -> BusCreator/24
  Subsystem20/1(Out1) -> BusCreator/23
  Subsystem27/1(Out1) -> BusCreator/22
  Subsystem26/1(Out1) -> BusCreator/21
  BusCreator/1 -> TimeStamp/1
  Subsystem4/1(Out1) -> BusCreator/1
  Subsystem5/1(Out1) -> BusCreator/2
  Subsystem6/1(Out1) -> BusCreator/3
  Subsystem7/1(Out1) -> BusCreator/4
  Subsystem8/1(Out1) -> BusCreator/5
  Subsystem9/1(Out1) -> BusCreator/6
  Subsystem10/1(Out1) -> BusCreator/7
  Subsystem11/1(Out1) -> BusCreator/8
  Subsystem14/1(Out1) -> BusCreator/9
  Subsystem15/1(Out1) -> BusCreator/10
  Subsystem16/1(Out1) -> BusCreator/11
  Subsystem17/1(Out1) -> BusCreator/12
  Subsystem18/1(Out1) -> BusCreator/13
  Subsystem19/1(Out1) -> BusCreator/14
  Subsystem12/1(Out1) -> BusCreator/15
  Subsystem13/1(Out1) -> BusCreator/16
  Subsystem22/1(Out1) -> BusCreator/17
  Subsystem23/1(Out1) -> BusCreator/18
  Subsystem24/1(Out1) -> BusCreator/19
  Subsystem25/1(Out1) -> BusCreator/20

== system MIL4L3_SW6_V1_20220211/CarMaker/VehicleControl/Data Inport/SDFA-L3/Subsystem41 ==
  Bus Creator : BusCreator  Inputs=20
  Ground{,1..15} (16 alike) : Ground
  Subsystem : Subsystem
  Subsystem1 : Subsystem
  Subsystem2 : Subsystem
  Subsystem3 : Subsystem
  camera_timestamp : Outport
  wires:
  Ground15/1 -> Bus Creator/20
  Ground14/1 -> Bus Creator/19
  Ground13/1 -> Bus Creator/18
  Ground12/1 -> Bus Creator/17
  Ground11/1 -> Bus Creator/16
  Ground10/1 -> Bus Creator/15
  Ground9/1 -> Bus Creator/14
  Ground8/1 -> Bus Creator/13
  Ground7/1 -> Bus Creator/12
  Ground6/1 -> Bus Creator/11
  Ground5/1 -> Bus Creator/10
  Ground4/1 -> Bus Creator/9
  Ground3/1 -> Bus Creator/8
  Ground2/1 -> Bus Creator/7
  Ground1/1 -> Bus Creator/6
  Ground/1 -> Bus Creator/5
  Subsystem3/1(camera_timestamp) -> Bus Creator/4
  Subsystem2/1(camera_timestamp) -> Bus Creator/3
  Subsystem1/1(camera_timestamp) -> Bus Creator/2
  Subsystem/1(camera_timestamp) -> Bus Creator/1
  Bus Creator/1 -> camera_timestamp/1

== system MIL4L3_SW6_V1_20220211/CarMaker/VehicleControl/Data Inport/SDFA-L3/Subsystem46 ==
  BusCreator : BusCreator  Inputs=10
  Data Type Conversion{1..3,89} (4 alike) : DataTypeConversion  OutDataTypeStr=uint16
  Ground{,1..5} (6 alike) : Ground
  Read CM Dict1 : CarMaker4SL/Read CM Dict  xname=User.IO.Out.Id_S2_002  xsync=off
  Read CM Dict2 : CarMaker4SL/Read CM Dict  xname=User.IO.Out.Id_S2_003  xsync=off
  Read CM Dict3 : CarMaker4SL/Read CM Dict  xname=User.IO.Out.Id_S2_004  xsync=off
  Read CM Dict5 : CarMaker4SL/Read CM Dict  xname=User.IO.Out.Id_S2_001  xsync=off
  LFtar_id : Outport
  wires:
  Data Type Conversion3/1 -> BusCreator/4
  Data Type Conversion2/1 -> BusCreator/3
  Data Type Conversion1/1 -> BusCreator/2
  Data Type Conversion89/1 -> BusCreator/1
  Read CM Dict3/1 -> Data Type Conversion3/1
  Read CM Dict2/1 -> Data Type Conversion2/1
  Read CM Dict1/1 -> Data Type Conversion1/1
  Read CM Dict5/1 -> Data Type Conversion89/1
  Ground5/1 -> BusCreator/10
  Ground4/1 -> BusCreator/9
  Ground3/1 -> BusCreator/8
  Ground2/1 -> BusCreator/7
  Ground1/1 -> BusCreator/6
  Ground/1 -> BusCreator/5
  BusCreator/1 -> LFtar_id/1

== system MIL4L3_SW6_V1_20220211/CarMaker/VehicleControl/Data Inport/SDFA-L3/Subsystem47 ==
  BusCreator : BusCreator  Inputs=10
  Data Type Conversion{1..3,91} (4 alike) : DataTypeConversion  OutDataTypeStr=single
  Ground{,1..5} (6 alike) : Ground
  Read CM Dict1 : CarMaker4SL/Read CM Dict  xname=User.IO.Out.XPos_S2_002  xsync=off
  Read CM Dict2 : CarMaker4SL/Read CM Dict  xname=User.IO.Out.XPos_S2_003  xsync=off
  Read CM Dict3 : CarMaker4SL/Read CM Dict  xname=User.IO.Out.XPos_S2_004  xsync=off
  Read CM Dict5 : CarMaker4SL/Read CM Dict  xname=User.IO.Out.XPos_S2_001  xsync=off
  LFtar_Xpos : Outport
  wires:
  Data Type Conversion3/1 -> BusCreator/4
  Data Type Conversion2/1 -> BusCreator/3
  Data Type Conversion1/1 -> BusCreator/2
  Data Type Conversion91/1 -> BusCreator/1
  BusCreator/1 -> LFtar_Xpos/1
  Read CM Dict3/1 -> Data Type Conversion3/1
  Read CM Dict2/1 -> Data Type Conversion2/1
  Read CM Dict1/1 -> Data Type Conversion1/1
  Read CM Dict5/1 -> Data Type Conversion91/1
  Ground/1 -> BusCreator/5
  Ground1/1 -> BusCreator/6
  Ground2/1 -> BusCreator/7
  Ground3/1 -> BusCreator/8
  Ground4/1 -> BusCreator/9
  Ground5/1 -> BusCreator/10

== system MIL4L3_SW6_V1_20220211/CarMaker/VehicleControl/Data Inport/SDFA-L3/Subsystem48 ==
  BusCreator : BusCreator  Inputs=10
  Data Type Conversion{1..3,92} (4 alike) : DataTypeConversion  OutDataTypeStr=single
  Ground{,1..5} (6 alike) : Ground
  Read CM Dict1 : CarMaker4SL/Read CM Dict  xname=User.IO.Out.YPos_S2_002  xsync=off
  Read CM Dict2 : CarMaker4SL/Read CM Dict  xname=User.IO.Out.YPos_S2_003  xsync=off
  Read CM Dict3 : CarMaker4SL/Read CM Dict  xname=User.IO.Out.YPos_S2_004  xsync=off
  Read CM Dict5 : CarMaker4SL/Read CM Dict  xname=User.IO.Out.YPos_S2_001  xsync=off
  LFtar_Ypos : Outport
  wires:
  Data Type Conversion3/1 -> BusCreator/4
  Data Type Conversion2/1 -> BusCreator/3
  Data Type Conversion1/1 -> BusCreator/2
  Data Type Conversion92/1 -> BusCreator/1
  Ground5/1 -> BusCreator/10
  Ground4/1 -> BusCreator/9
  Ground3/1 -> BusCreator/8
  Ground2/1 -> BusCreator/7
  Ground1/1 -> BusCreator/6
  Ground/1 -> BusCreator/5
  Read CM Dict5/1 -> Data Type Conversion92/1
  Read CM Dict1/1 -> Data Type Conversion1/1
  Read CM Dict2/1 -> Data Type Conversion2/1
  Read CM Dict3/1 -> Data Type Conversion3/1
  BusCreator/1 -> LFtar_Ypos/1

== system MIL4L3_SW6_V1_20220211/CarMaker/VehicleControl/Data Inport/SDFA-L3/Subsystem49 ==
  BusCreator : BusCreator  Inputs=10
  Data Type Conversion{1..3,92} (4 alike) : DataTypeConversion  OutDataTypeStr=single
  Ground{,1..5} (6 alike) : Ground
  Read CM Dict1 : CarMaker4SL/Read CM Dict  xname=User.IO.Out.XVelocity_S2_002  xsync=off
  Read CM Dict2 : CarMaker4SL/Read CM Dict  xname=User.IO.Out.XVelocity_S2_003  xsync=off
  Read CM Dict3 : CarMaker4SL/Read CM Dict  xname=User.IO.Out.XVelocity_S2_004  xsync=off
  Read CM Dict5 : CarMaker4SL/Read CM Dict  xname=User.IO.Out.XVelocity_S2_001  xsync=off
  LFtar_Xvelocity : Outport
  wires:
  Data Type Conversion3/1 -> BusCreator/4
  Data Type Conversion2/1 -> BusCreator/3
  Data Type Conversion1/1 -> BusCreator/2
  Data Type Conversion92/1 -> BusCreator/1
  BusCreator/1 -> LFtar_Xvelocity/1
  Read CM Dict3/1 -> Data Type Conversion3/1
  Read CM Dict2/1 -> Data Type Conversion2/1
  Read CM Dict1/1 -> Data Type Conversion1/1
  Read CM Dict5/1 -> Data Type Conversion92/1
  Ground/1 -> BusCreator/5
  Ground1/1 -> BusCreator/6
  Ground2/1 -> BusCreator/7
  Ground3/1 -> BusCreator/8
  Ground4/1 -> BusCreator/9
  Ground5/1 -> BusCreator/10

== system MIL4L3_SW6_V1_20220211/CarMaker/VehicleControl/Data Inport/SDFA-L3/Subsystem5 ==
  Bus Creator : BusCreator  Inputs=20
  Ground{,1..15} (16 alike) : Ground
  Read CM Dict : CarMaker4SL/Read CM Dict  xname=User.IO.Out.IFC_obj01_BrakeLight  xsync=off
  Read CM Dict1 : CarMaker4SL/Read CM Dict  xname=User.IO.Out.IFC_obj02_BrakeLight  xsync=off
  Read CM Dict2 : CarMaker4SL/Read CM Dict  xname=User.IO.Out.IFC_obj03_BrakeLight  xsync=off
  Read CM Dict3 : CarMaker4SL/Read CM Dict  xname=User.IO.Out.IFC_obj04_BrakeLight  xsync=off
  obj_BrakeLight : Outport
  wires:
  Read CM Dict2/1 -> Bus Creator/3
  Ground8/1 -> Bus Creator/13
  Ground5/1 -> Bus Creator/10
  Ground9/1 -> Bus Creator/14
  Ground4/1 -> Bus Creator/9
  Read CM Dict3/1 -> Bus Creator/4
  Ground7/1 -> Bus Creator/12
  Ground/1 -> Bus Creator/5
  Ground2/1 -> Bus Creator/7
  Ground13/1 -> Bus Creator/18
  Ground10/1 -> Bus Creator/15
  Ground6/1 -> Bus Creator/11
  Read CM Dict/1 -> Bus Creator/1
  Read CM Dict1/1 -> Bus Creator/2
  Ground1/1 -> Bus Creator/6
  Ground3/1 -> Bus Creator/8
  Ground12/1 -> Bus Creator/17
  Ground14/1 -> Bus Creator/19
  Ground11/1 -> Bus Creator/16
  Ground15/1 -> Bus Creator/20
  Bus Creator/1 -> obj_BrakeLight/1

== system MIL4L3_SW6_V1_20220211/CarMaker/VehicleControl/Data Inport/SDFA-L3/Subsystem50 ==
  BusCreator : BusCreator  Inputs=10
  Data Type Conversion{1..3,92} (4 alike) : DataTypeConversion  OutDataTypeStr=single
  Ground{,1..5} (6 alike) : Ground
  Read CM Dict1 : CarMaker4SL/Read CM Dict  xname=User.IO.Out.YVelocity_S2_002  xsync=off
  Read CM Dict2 : CarMaker4SL/Read CM Dict  xname=User.IO.Out.YVelocity_S2_003  xsync=off
  Read CM Dict3 : CarMaker4SL/Read CM Dict  xname=User.IO.Out.YVelocity_S2_004  xsync=off
  Read CM Dict5 : CarMaker4SL/Read CM Dict  xname=User.IO.Out.YVelocity_S2_001  xsync=off
  LFtar_Yvelocity : Outport
  wires:
  Data Type Conversion92/1 -> BusCreator/1
  Data Type Conversion2/1 -> BusCreator/3
  Data Type Conversion3/1 -> BusCreator/4
  Data Type Conversion1/1 -> BusCreator/2
  Ground5/1 -> BusCreator/10
  Ground4/1 -> BusCreator/9
  Ground3/1 -> BusCreator/8
  Ground2/1 -> BusCreator/7
  Ground1/1 -> BusCreator/6
  Ground/1 -> BusCreator/5
  Read CM Dict5/1 -> Data Type Conversion92/1
  Read CM Dict1/1 -> Data Type Conversion1/1
  Read CM Dict2/1 -> Data Type Conversion2/1
  Read CM Dict3/1 -> Data Type Conversion3/1
  BusCreator/1 -> LFtar_Yvelocity/1

== system MIL4L3_SW6_V1_20220211/CarMaker/VehicleControl/Data Inport/SDFA-L3/Subsystem51 ==
  BusCreator : BusCreator  Inputs=10
  Data Type Conversion{1..3,92} (4 alike) : DataTypeConversion  OutDataTypeStr=single
  Ground{,1..5} (6 alike) : Ground
  Read CM Dict1 : CarMaker4SL/Read CM Dict  xname=User.IO.Out.XAcceleration_S2_002  xsync=off
  Read CM Dict2 : CarMaker4SL/Read CM Dict  xname=User.IO.Out.XAcceleration_S2_003  xsync=off
  Read CM Dict3 : CarMaker4SL/Read CM Dict  xname=User.IO.Out.XAcceleration_S2_004  xsync=off
  Read CM Dict5 : CarMaker4SL/Read CM Dict  xname=User.IO.Out.XAcceleration_S2_001  xsync=off
  LFtar_Xacceleration : Outport
  wires:
  Data Type Conversion1/1 -> BusCreator/2
  Data Type Conversion2/1 -> BusCreator/3
  Data Type Conversion3/1 -> BusCreator/4
  Data Type Conversion92/1 -> BusCreator/1
  BusCreator/1 -> LFtar_Xacceleration/1
  Read CM Dict3/1 -> Data Type Conversion3/1
  Read CM Dict2/1 -> Data Type Conversion2/1
  Read CM Dict1/1 -> Data Type Conversion1/1
  Read CM Dict5/1 -> Data Type Conversion92/1
  Ground/1 -> BusCreator/5
  Ground1/1 -> BusCreator/6
  Ground2/1 -> BusCreator/7
  Ground3/1 -> BusCreator/8
  Ground4/1 -> BusCreator/9
  Ground5/1 -> BusCreator/10

== system MIL4L3_SW6_V1_20220211/CarMaker/VehicleControl/Data Inport/SDFA-L3/Subsystem52 ==
  BusCreator : BusCreator  Inputs=10
  Data Type Conversion{1..3,92} (4 alike) : DataTypeConversion  OutDataTypeStr=single
  Ground{,1..5} (6 alike) : Ground
  Read CM Dict1 : CarMaker4SL/Read CM Dict  xname=User.IO.Out.YAcceleration_S2_002  xsync=off
  Read CM Dict2 : CarMaker4SL/Read CM Dict  xname=User.IO.Out.YAcceleration_S2_003  xsync=off
  Read CM Dict3 : CarMaker4SL/Read CM Dict  xname=User.IO.Out.YAcceleration_S2_004  xsync=off
  Read CM Dict5 : CarMaker4SL/Read CM Dict  xname=User.IO.Out.YAcceleration_S2_001  xsync=off
  LFtar_Yacceleration : Outport
  wires:
  Data Type Conversion2/1 -> BusCreator/3
  Data Type Conversion3/1 -> BusCreator/4
  Data Type Conversion92/1 -> BusCreator/1
  Data Type Conversion1/1 -> BusCreator/2
  Ground5/1 -> BusCreator/10
  Ground4/1 -> BusCreator/9
  Ground3/1 -> BusCreator/8
  Ground2/1 -> BusCreator/7
  Ground1/1 -> BusCreator/6
  Ground/1 -> BusCreator/5
  Read CM Dict5/1 -> Data Type Conversion92/1
  Read CM Dict1/1 -> Data Type Conversion1/1
  Read CM Dict2/1 -> Data Type Conversion2/1
  Read CM Dict3/1 -> Data Type Conversion3/1
  BusCreator/1 -> LFtar_Yacceleration/1

== system MIL4L3_SW6_V1_20220211/CarMaker/VehicleControl/Data Inport/SDFA-L3/Subsystem53 ==
  BusCreator : BusCreator  Inputs=10
  Data Type Conversion{1..3,92} (4 alike) : DataTypeConversion  OutDataTypeStr=single
  Ground{,1..5} (6 alike) : Ground
  Read CM Dict1 : CarMaker4SL/Read CM Dict  xname=User.IO.Out.Width_S2_002  xsync=off
  Read CM Dict2 : CarMaker4SL/Read CM Dict  xname=User.IO.Out.Width_S2_003  xsync=off
  Read CM Dict3 : CarMaker4SL/Read CM Dict  xname=User.IO.Out.Width_S2_004  xsync=off
  Read CM Dict5 : CarMaker4SL/Read CM Dict  xname=User.IO.Out.Width_S2_001  xsync=off
  LFtar_Width : Outport
  wires:
  Data Type Conversion92/1 -> BusCreator/1
  Data Type Conversion3/1 -> BusCreator/4
  Data Type Conversion2/1 -> BusCreator/3
  Data Type Conversion1/1 -> BusCreator/2
  BusCreator/1 -> LFtar_Width/1
  Read CM Dict3/1 -> Data Type Conversion3/1
  Read CM Dict2/1 -> Data Type Conversion2/1
  Read CM Dict1/1 -> Data Type Conversion1/1
  Read CM Dict5/1 -> Data Type Conversion92/1
  Ground/1 -> BusCreator/5
  Ground1/1 -> BusCreator/6
  Ground2/1 -> BusCreator/7
  Ground3/1 -> BusCreator/8
  Ground4/1 -> BusCreator/9
  Ground5/1 -> BusCreator/10

== system MIL4L3_SW6_V1_20220211/CarMaker/VehicleControl/Data Inport/SDFA-L3/Subsystem54 ==
  BusCreator : BusCreator  Inputs=10
  Data Type Conversion{1..3,92} (4 alike) : DataTypeConversion  OutDataTypeStr=single
  Ground{,1..5} (6 alike) : Ground
  Read CM Dict1 : CarMaker4SL/Read CM Dict  xname=User.IO.Out.Length_S2_002  xsync=off
  Read CM Dict2 : CarMaker4SL/Read CM Dict  xname=User.IO.Out.Length_S2_003  xsync=off
  Read CM Dict3 : CarMaker4SL/Read CM Dict  xname=User.IO.Out.Length_S2_004  xsync=off
  Read CM Dict5 : CarMaker4SL/Read CM Dict  xname=User.IO.Out.Length_S2_001  xsync=off
  LFtar_Length : Outport
  wires:
  Data Type Conversion2/1 -> BusCreator/3
  Data Type Conversion92/1 -> BusCreator/1
  Data Type Conversion3/1 -> BusCreator/4
  Data Type Conversion1/1 -> BusCreator/2
  Ground5/1 -> BusCreator/10
  Ground4/1 -> BusCreator/9
  Ground3/1 -> BusCreator/8
  Ground2/1 -> BusCreator/7
  Ground1/1 -> BusCreator/6
  Ground/1 -> BusCreator/5
  Read CM Dict5/1 -> Data Type Conversion92/1
  Read CM Dict1/1 -> Data Type Conversion1/1
  Read CM Dict2/1 -> Data Type Conversion2/1
  Read CM Dict3/1 -> Data Type Conversion3/1
  BusCreator/1 -> LFtar_Length/1

== system MIL4L3_SW6_V1_20220211/CarMaker/VehicleControl/Data Inport/SDFA-L3/Subsystem55 ==
  BusCreator : BusCreator  Inputs=10
  Data Type Conversion{1..3,92} (4 alike) : DataTypeConversion  OutDataTypeStr=single
  Ground{,1..5} (6 alike) : Ground
  Read CM Dict1 : CarMaker4SL/Read CM Dict  xname=User.IO.Out.Orientation_S2_002  xsync=off
  Read CM Dict2 : CarMaker4SL/Read CM Dict  xname=User.IO.Out.Orientation_S2_003  xsync=off
  Read CM Dict3 : CarMaker4SL/Read CM Dict  xname=User.IO.Out.Orientation_S2_004  xsync=off
  Read CM Dict5 : CarMaker4SL/Read CM Dict  xname=User.IO.Out.Orientation_S2_001  xsync=off
  LFtar_Orientation : Outport
  wires:
  Data Type Conversion3/1 -> BusCreator/4
  Data Type Conversion92/1 -> BusCreator/1
  Data Type Conversion2/1 -> BusCreator/3
  Data Type Conversion1/1 -> BusCreator/2
  BusCreator/1 -> LFtar_Orientation/1
  Read CM Dict3/1 -> Data Type Conversion3/1
  Read CM Dict2/1 -> Data Type Conversion2/1
  Read CM Dict1/1 -> Data Type Conversion1/1
  Read CM Dict5/1 -> Data Type Conversion92/1
  Ground/1 -> BusCreator/5
  Ground1/1 -> BusCreator/6
  Ground2/1 -> BusCreator/7
  Ground3/1 -> BusCreator/8
  Ground4/1 -> BusCreator/9
  Ground5/1 -> BusCreator/10

== system MIL4L3_SW6_V1_20220211/CarMaker/VehicleControl/Data Inport/SDFA-L3/Subsystem56 ==
  BusCreator : BusCreator  Inputs=10
  Data Type Conversion{1..3,92} (4 alike) : DataTypeConversion  OutDataTypeStr=single
  Ground{,1..5} (6 alike) : Ground
  Read CM Dict1 : CarMaker4SL/Read CM Dict  xname=User.IO.Out.ExistenceProbability_S2_002  xsync=off
  Read CM Dict2 : CarMaker4SL/Read CM Dict  xname=User.IO.Out.ExistenceProbability_S2_003  xsync=off
  Read CM Dict3 : CarMaker4SL/Read CM Dict  xname=User.IO.Out.ExistenceProbability_S2_004  xsync=off
  Read CM Dict5 : CarMaker4SL/Read CM Dict  xname=User.IO.Out.ExistenceProbability_S2_001  xsync=off
  LFtar_ExistenceProbability : Outport
  wires:
  Data Type Conversion2/1 -> BusCreator/3
  Data Type Conversion92/1 -> BusCreator/1
  Data Type Conversion3/1 -> BusCreator/4
  Data Type Conversion1/1 -> BusCreator/2
  Ground5/1 -> BusCreator/10
  Ground4/1 -> BusCreator/9
  Ground3/1 -> BusCreator/8
  Ground2/1 -> BusCreator/7
  Ground1/1 -> BusCreator/6
  Ground/1 -> BusCreator/5
  Read CM Dict5/1 -> Data Type Conversion92/1
  Read CM Dict1/1 -> Data Type Conversion1/1
  Read CM Dict2/1 -> Data Type Conversion2/1
  Read CM Dict3/1 -> Data Type Conversion3/1
  BusCreator/1 -> LFtar_ExistenceProbability/1

== system MIL4L3_SW6_V1_20220211/CarMaker/VehicleControl/Data Inport/SDFA-L3/Subsystem57 ==
  BusCreator : BusCreator  Inputs=10
  Data Type Conversion{1..3,92} (4 alike) : DataTypeConversion  OutDataTypeStr=uint8
  Ground{,1..5} (6 alike) : Ground
  Read CM Dict1 : CarMaker4SL/Read CM Dict  xname=User.IO.Out.ClassHighest_S2_002  xsync=off
  Read CM Dict2 : CarMaker4SL/Read CM Dict  xname=User.IO.Out.ClassHighest_S2_003  xsync=off
  Read CM Dict3 : CarMaker4SL/Read CM Dict  xname=User.IO.Out.ClassHighest_S2_004  xsync=off
  Read CM Dict5 : CarMaker4SL/Read CM Dict  xname=User.IO.Out.ClassHighest_S2_001  xsync=off
  LFtar_Class : Outport
  wires:
  Data Type Conversion92/1 -> BusCreator/1
  Data Type Conversion3/1 -> BusCreator/4
  Data Type Conversion1/1 -> BusCreator/2
  Data Type Conversion2/1 -> BusCreator/3
  BusCreator/1 -> LFtar_Class/1
  Read CM Dict3/1 -> Data Type Conversion3/1
  Read CM Dict2/1 -> Data Type Conversion2/1
  Read CM Dict1/1 -> Data Type Conversion1/1
  Read CM Dict5/1 -> Data Type Conversion92/1
  Ground/1 -> BusCreator/5
  Ground1/1 -> BusCreator/6
  Ground2/1 -> BusCreator/7
  Ground3/1 -> BusCreator/8
  Ground4/1 -> BusCreator/9
  Ground5/1 -> BusCreator/10
